simulink model "Noa_Nofusion_angle"  (R2020b)
settings: Solver=FixedStepDiscrete  StartTime=0.0  StopTime=Inf  FixedStep=0.01  RelTol=1e-3
PostLoadFcn:
  | if any(exist('dsrtsu_mdlpostloadfcn', 'file') ~= 0), dsrtsu_mdlpostloadfcn('Execute', bdroot); end
InitFcn:
  | , if any(exist('rtifpga_mdlclblib', 'file') ~= 0), rtifpga_mdlclblib('Init', bdroot); end,
  | , if any(exist('dsmpb_private', 'file') ~= 0), dsmpb_private('dsmpb_mdlclblib', 'Init', bdroot); end,
undefined symbols (not defined in the file): ACC_TimeGap_DecSetSwt, ACC_TimeGap_IncSetSwt, AccelPedalPosn, AccelPedalPosnVldty, AccelPedlPosnDiagc, AccPedalOverride, ACU_ShiftInProgress, ADAS_Posn_CurLane, AESSwtReq, ALC_SwtReq, BrkPedalSts, CC_ACC_CANCEL_OFFSwt, CC_ACC_CRUISE_OFFSwt, CC_ACC_DecSetSpd_SetSwt, CC_ACC_IncSetSpd_ResuSwt, CC_ACCSwtErr, CharSpd_ms, CSA_NODE, CURRENT_GEAR, CurrentGearValid, DiscIntNeverNeededParam, DrvDoorSts, DrvSBR, DrvTrqReqOvld, ECMACCInterface, ECMRespACC, ELKSwtReq, EngLimpHomeSts, EngSpd, EngState, EngState_PHEV, EngTrqMaxActSpd, EngTrqMinAct, EPS_DrvInpTrqVal_HighReslolution, EPS_FailSts, EPS_LKATorqOvrlDlvd, EPS_LKATorqOvrlDlvdVld, EPS_LKATrqOvlDlvdSts, EPS_SteerMod, EPS_TrqSnsrSts, EQ4_APPINFO, EQ4_LA_ELEM, EQ4_LA_HDR, EQ4_LAP_ELEM, EQ4_LAP_HDR, EQ4_LH_ELEM, EQ4_LH_HDR, EQ4_LRE_ELEM, EQ4_LRE_HDR, ESS_PedSwtReq, ESS_VehSwtReq, FFogLmpSts_F_Pbox, FLWheelDriveDirection, FLWheelSpd, FrntWiprSwtSts, FrntWshrSwtSts, FRWheelDriveDirection, FRWheelSpd, HazardLmpSwtSts, HCU_AccelPedalPosn_Diag ... (+151)
libraries: simulink x138, dsmpblib x33, canfdmsglib x10
(part 17 of 17)

== matlab function Noa_Nofusion_angle/TOS2/Subsystem1/ACCOSM/HWA_Task100ms1/ACC_DisplayBar ==
  data: TimeGap input; DisplayBar output uint8; DesireDistance input; ACCmode input; TargetRange input; Scale input; TargetExist input; DisplayBarK1 input uint8
function DisplayBar = fcn(TimeGap,DesireDistance,ACCmode,TargetRange,Scale,TargetExist,DisplayBarK1)
%#codegen
DisplayBar = DisplayBarK1;

ScaleDis = Scale*DesireDistance;
upScaleDis = (Scale+single(0.05))*DesireDistance;
lowScaleDis = (Scale-single(0.05))*DesireDistance;

i = TimeGap;

if (ACCmode==0)||(ACCmode==7)
    DisplayBar = uint8(0);
else
    if TargetExist==false
        DisplayBar=uint8(0);
    else
        switch(DisplayBarK1)
            case uint8(0)
                 if TargetRange> ScaleDis(i,3)
                     DisplayBar=uint8(4);
                 else
                     if TargetRange>ScaleDis(i,2)
                         DisplayBar=uint8(3);
                     else
                         if TargetRange>ScaleDis(i,1)
                             DisplayBar=uint8(2);
                         else
                             DisplayBar=uint8(1);
                         end
                     end
                 end
            case uint8(1)
                 if TargetRange> upScaleDis(i,3)
                     DisplayBar=uint8(4);
                 else
                     if TargetRange>upScaleDis(i,2)
                         DisplayBar=uint8(3);
                     else
                         if TargetRange>upScaleDis(i,1)
                             DisplayBar=uint8(2);
                         else
                             DisplayBar=uint8(1);
                         end
                     end
                 end
            case uint8(2)
                 if TargetRange> upScaleDis(i,3)
                     DisplayBar=uint8(4);
                 else
                     if TargetRange>upScaleDis(i,2)
                         DisplayBar=uint8(3);
                     else
                         if TargetRange>lowScaleDis(i,1)
                             DisplayBar=uint8(2);
                         else
                             DisplayBar=uint8(1);
                         end
                     end
                 end   
            case uint8(3)
                 if TargetRange> upScaleDis(i,3)
                     DisplayBar=uint8(4);
                 else
                     if TargetRange>lowScaleDis(i,2)
                         DisplayBar=uint8(3);
                     else
                         if TargetRange>lowScaleDis(i,1)
                             DisplayBar=uint8(2);
                         else
                             DisplayBar=uint8(1);
                         end
                     end
                end
            case uint8(4)
                 if TargetRange> lowScaleDis(i,3)
                     DisplayBar=uint8(4);
                 else
                     if TargetRange>lowScaleDis(i,2)
                         DisplayBar=uint8(3);
                     else
                         if TargetRange>lowScaleDis(i,1)
                             DisplayBar=uint8(2);
                         else
                             DisplayBar=uint8(1);
                         end
                     end
                 end      
        end    
    end
end

== matlab function Noa_Nofusion_angle/TOS2/Subsystem1/ACCOSM/HWA_Task100ms1/Dyc ==
  data: kapTrajFiltK1 input single size=1; vRef input single size=1; kapTrajFilt output single size=1; kapCourseErr output single; kapTraj input single size=1; alpSideSlipAngle input single size=1; A2 input single size=1; A1 input single size=1; LineValid input boolean size=1; ObjDx input single size=15; ObjDy input single size=15; TarLineValid input boolean; TarLineA2 input single; TarLineA1 input single; TarLineA0 input single size=1; dxC0 output single size=1; aPC0 output single size=1; bPC0 output single size=1; cPC0 output single size=1; aPC1 output single size=1; bPC1 output single size=1; cPC1 output single size=1; ObjDyc output single size=15
function [kapTrajFilt,kapCourseErr,dxC0,aPC0,bPC0,cPC0,aPC1,bPC1,cPC1,ObjDyc] = ...
    DriveCourseCalc(kapTrajFiltK1,vRef,kapTraj,alpSideSlipAngle,...
    A2,A1,LineValid,ObjDx,ObjDy,TarLineValid,TarLineA2,TarLineA1,TarLineA0)

ObjDyc = single(zeros(15,1));

if vRef>8.33
    t_alpSideSlipAngle = -alpSideSlipAngle;
else
    t_alpSideSlipAngle = single(0);
end

temp1 = single(0.1)/(single(0.1) + interpolate(single(24),single(0),single(55),single(0.4),vRef));

kapTrajFilt = kapTrajFiltK1 + temp1*(kapTraj - kapTrajFiltK1);

temp1 = abs(kapTraj*vRef);

if (temp1<0.001)&&(vRef>8.3)
    t_kapTrajwHyst = single(0);
else
    t_kapTrajwHyst = kapTrajFilt;
end

if TarLineValid
    temp = interpolate(single(0.2),single(0.2),single(1.5),single(1),abs(TarLineA0));
    dxC0Min = single(3);
else
    temp = single(1);
    dxC0Min = single(10);
end

dxC0 = max(vRef*temp,dxC0Min);
aPC0 = 0.5*t_kapTrajwHyst*(single(1)+1.5*t_alpSideSlipAngle*t_alpSideSlipAngle);
bPC0 = t_alpSideSlipAngle;
cPC0 = single(0);

temp1 = single(0.1)*abs(t_kapTrajwHyst);
temp2 = min(single(0.00013),single(0.004)/max(vRef,single(10)));
kapCourseErr = max(temp1,temp2);

aPC1 = aPC0;
bPC1 = bPC0;
cPC1 = single(0);

Low = interpolate(single(4),single(1),single(20),single(0),abs(atan(A1)));    % low vehiclespeed lanechange Angle is 4deg~20deg;
High = interpolate(single(4),single(1),single(10),single(0),abs(atan(A1)));   % low vehiclespeed lanechange Angle is 4deg~10deg;
t_vRefFactor = interpolate(single(5),Low,single(25),High,vRef);

t_Factor = single(1)*t_vRefFactor;

if TarLineValid==true
    aPC1 = TarLineA2;
    bPC1 = TarLineA1;
    cPC1 = (aPC0 - aPC1)*dxC0*dxC0 + (bPC0 - bPC1)*dxC0;
else
    if LineValid
        aPC1 = aPC0*(1 - t_Factor) + A2*t_Factor;
        bPC1 = bPC0*(1 - t_Factor) + A1*t_Factor;
        cPC1 = (aPC0 - aPC1)*dxC0*dxC0 + (bPC0 - bPC1)*dxC0;
    end
end

for i=1:15
   if ObjDx(i)>dxC0
      ObjDyc(i) =  ObjDy(i) - (aPC1*ObjDx(i)*ObjDx(i) + bPC1*ObjDx(i) + cPC1);
   else
      ObjDyc(i) =  ObjDy(i) - (aPC0*ObjDx(i)*ObjDx(i) + bPC0*ObjDx(i));
   end
end
end


function out = interpolate(x1,z1,x2,z2,Raw)
if Raw<=x1
    out = z1;
else
    if Raw>=x2
        out = z2;
    else
        out = z1 + (Raw-x1)*(z2-z1)/(x2-x1);
    end
end
end

== matlab function Noa_Nofusion_angle/TOS2/Subsystem1/ACCOSM/HWA_Task100ms1/DycCutIn ==
  data: ObjValid input boolean size=15; ObjDyc input single size=15; ObjMoveSts input uint8 size=15; ObjDycCutIn output single size=15; ObjMove_b output boolean size=15; ObjCnt input uint8 size=15; ObjDycHist input single size=15; ObjqDycHist input single size=15; dycFiltK1 input single size=15; ObjDycFilt output single size=15
function [ObjDycCutIn,ObjMove_b,ObjDycFilt] = ...
    ObjDycCutInCalc(ObjValid,ObjDyc,ObjMoveSts,ObjCnt,ObjDycHist,ObjqDycHist,dycFiltK1)
 
ObjDycCutIn = single(zeros(15,1));
ObjDycFilt = single(zeros(15,1));
ObjMove_b = false(15,1); 
 
for i=1:15
    if ObjValid(i)
        t_dyc = ObjDyc(i);
        t_dycHist = ObjDycHist(i);
        t_qDycHist = ObjqDycHist(i);
        
        weightDycHist = t_qDycHist*0.1;
        weightDyc = single(1) - weightDycHist;
        
        t_dycASI = weightDycHist*t_dycHist + weightDyc*t_dyc;
        ObjDycCutIn(i) = t_dycASI;
        
        if ObjCnt(i)>2
            ObjDycFilt(i) = 0.028*(t_dycASI - dycFiltK1(i)) + dycFiltK1(i);
        else
            ObjDycFilt(i) = t_dycASI;
        end
        if ObjMoveSts(i)==2
            ObjMove_b(i) = true;
        end
    end
end

== matlab function Noa_Nofusion_angle/TOS2/Subsystem1/ACCOSM/HWA_Task100ms1/DycHistCalc ==
  data: TrajHistBufferBTrajEnd input boolean; ObjTrajNumber input uint8; ObjDycHist output single; TrajCurrentIndex input uint8; TrajHistBufferBValid input boolean; TrajHistBufferDxv input single; TrajHistBufferDyv input single; ObjValid input boolean; ObjqDycHist output single; dxC0 input; aP0 input; bP0 input; cP0 input; aP1 input; bP1 input; cP1 input
function [ObjDycHist,ObjqDycHist] = DycHistCalc(TrajHistBufferBTrajEnd,ObjTrajNumber,TrajCurrentIndex,...
    TrajHistBufferBValid,TrajHistBufferDxv,TrajHistBufferDyv,ObjValid,dxC0,aP0,bP0,cP0,aP1,bP1,cP1)

t_dxv = single(0);
t_dyv = single(0);
t_dxvK1 = single(0);
t_dyvK1 = single(0);
ObjDycHist = single(zeros(15,1));
ObjqDycHist = single(zeros(15,1));

for iObj=1:15
    t_TrajNumber = ObjTrajNumber(iObj);
    if t_TrajNumber<21
        t_End = false;
        t_Failed = false;
        t_TrajCurrentIndex = TrajCurrentIndex(t_TrajNumber);
        t_TrajEnd = TrajHistBufferBTrajEnd(t_TrajNumber,t_TrajCurrentIndex);
        if (ObjValid(iObj)==true)&&(t_TrajEnd==false)
            for k=1:24
                if t_End==false
                    if t_TrajCurrentIndex<k
                        t_Index = t_TrajCurrentIndex + uint8(25) - k;
                    else
                        t_Index = t_TrajCurrentIndex - k + uint8(1);
                    end
                    if t_Index==1
                        t_IndexK1 = uint8(24);
                    else
                        t_IndexK1 = t_Index - uint8(1);
                    end
                    t_ValidK1 = TrajHistBufferBValid(t_TrajNumber,t_IndexK1);
                    t_TrajEndK1 = TrajHistBufferBTrajEnd(t_TrajNumber,t_IndexK1);
                    t_dxv = TrajHistBufferDxv(t_TrajNumber,t_Index);
                    t_dxvK1 = TrajHistBufferDxv(t_TrajNumber,t_IndexK1);
                    t_dyv = TrajHistBufferDyv(t_TrajNumber,t_Index);
                    t_dyvK1 = TrajHistBufferDyv(t_TrajNumber,t_IndexK1);
                    
                    if (t_TrajEndK1==true)||(t_ValidK1==false)
                        t_End = true;
                        t_Failed = true;
                    end
                    if (t_dxv>=0)&&(t_dxvK1<=0)
                        t_End = true;
                    end
                end
            end
        end
        if (t_End==true)&&(t_Failed==false)
            if (t_dxv==t_dxvK1)
                t_dycHist = t_dyv;
            else
                t_dycHist = t_dyv - t_dxv*(t_dyvK1 - t_dyv)/(t_dxvK1 - t_dxv);
            end
            t_qDycHist = single(1);  
        else
            if (t_End==true)&&(t_Failed==true)&&(t_dxv>0)
                if t_dxv>(dxC0)
                    t_dycHist = t_dyv - (aP1*t_dxv*t_dxv + bP1*t_dxv + cP1); 
                else
                    t_dycHist = t_dyv - (aP0*t_dxv*t_dxv + bP0*t_dxv + cP0); 
                end
               t_qDycHist = max((single(80) - t_dxv)/single(80),single(0));
            else
                t_dycHist = single(0);
                t_qDycHist = single(0);
            end
        end
    else
        t_dycHist = single(0);
        t_qDycHist = single(0);
    end
    ObjDycHist(iObj) = t_dycHist;
    ObjqDycHist(iObj) = t_qDycHist;
end

== matlab function Noa_Nofusion_angle/TOS2/Subsystem1/ACCOSM/HWA_Task100ms1/LostTargetCalc ==
  data: ObjValid input boolean size=15; ReID output uint8 size=1; ObjDx input single size=15; ObjDy input single size=15; DeltaDx input single size=1; DeltaDy input single size=1; P0IDK1 input uint8 size=1; P0VxK1 input single size=1; P0DxK1 input single size=1; P0DyK1 input single size=1; P0RangeK1 input; P0ArGK1 input; P0DycK1 input single size=1; P0VycK1 input single size=1; P0CutIn_bK1 input boolean size=1; tTargetLostK1 input single size=1; ReRange output single size=1; ReArG output single size=1; ReDx output single size=1; ReDy output single size=1; ReVx output single size=1; ReCutIn_b output boolean size=1; ReDyc output single size=1; ReVyc output single size=1; TargetLost_b output boolean size=1; Covered_b output boolean size=1; tTargetLost output single size=1
function [ReID,ReRange,ReArG,ReDx,ReDy,ReVx,ReCutIn_b,ReDyc,ReVyc,TargetLost_b,Covered_b,tTargetLost]...
    = LostTargetCalc(ObjValid,ObjDx,ObjDy,DeltaDx,DeltaDy,...
    P0IDK1,P0VxK1,P0DxK1,P0DyK1,P0RangeK1,P0ArGK1,P0DycK1,P0VycK1,P0CutIn_bK1,tTargetLostK1)
 
ReID = P0IDK1;
ReRange = single(255);
ReArG = single(0);
ReDx = single(255);
ReDy = single(0);
ReVx = single(0);
ReDyc = single(0);
ReVyc = single(0);
ReCutIn_b = false;
TargetLost_b = false;
tTargetLost = single(0);
Covered_b = false;
 
if (P0IDK1>0)&&(P0IDK1<100)    % k1 Exist Target
    if ObjValid(P0IDK1)==false
        ExistNearObj = false;
        P0DxPred = P0DxK1 + 0.1*P0VxK1;
        P0DyPred = P0DyK1;
        P0RangePred = P0RangeK1 + 0.1*P0VxK1; 
        for i=1:15
            if (ObjValid(i)==true)&&(ObjDx(i)<P0DxPred)
                Covered_b = CoveredCalc(P0DxPred,P0DyPred,ObjDx(i),ObjDy(i),single(2.1),single(-0.1));
                if Covered_b==true
                   break; 
                end
            end
            if (ObjValid(i)==1)&&(abs(ObjDx(i)-P0DxPred)<DeltaDx)&&(abs(ObjDy(i)-P0DyPred)<DeltaDy)
               ExistNearObj = true;
               ReID = uint8(i);
               ReDx = ObjDx(i);
            end
        end
        if (ExistNearObj==false)&&(Covered_b==false)
            TargetLost_b = true;
            tTargetLost = single(0.1);
            ReID = uint8(255);
            ReRange = P0RangePred;
            ReArG = P0ArGK1;
            ReDx = P0DxPred;
            ReDy = P0DyPred;
            ReVx = P0VxK1;
            ReCutIn_b = P0CutIn_bK1;
            ReVyc = P0VycK1;
            ReDyc = P0DycK1 + 0.1*P0VycK1;
        end
    end
else
    if P0IDK1>100   %  k1 Exist Target Re
        ExistNearObj = false;
        P0DxPred = P0DxK1 + 0.1*P0VxK1;
        P0DyPred = P0DyK1;
        P0RangePred = P0RangeK1 + 0.1*P0VxK1; 

        for i=1:15
            if (ObjValid(i)==1)&&(abs(ObjDx(i)-P0DxPred)<DeltaDx)&&(abs(ObjDy(i)-P0DyPred)<DeltaDy)
                ExistNearObj = true;
                ReID = uint8(i);
                ReDx = ObjDx(i);
                TargetLost_b = false;
                tTargetLost = single(0);
            end
        end
        if ExistNearObj==false
            TargetLost_b = true;
            tTargetLost = tTargetLostK1 + single(0.1);
            ReID = uint8(255);
            ReRange = P0RangePred;
            ReArG = P0ArGK1;
            ReDx = P0DxPred;
            ReDy = P0DyPred;
            ReVx = P0VxK1;
            ReCutIn_b = P0CutIn_bK1;
            ReVyc = P0VycK1;
            ReDyc = P0DycK1 + 0.1*P0VycK1;
        end
    end
end
end
 
function t_Covered_b = CoveredCalc(DxPred,DyPred,Dx,Dy,IFVDx,IFVDy)
y = (IFVDy - DyPred)*(Dx - DxPred)/(IFVDx - DxPred) + DyPred ;
Delta = single(0.8) + (Dx - IFVDx)/(DxPred - IFVDx);
if abs(Dy - y)<=Delta
    t_Covered_b = true;
else
    t_Covered_b = false;
end
end

== matlab function Noa_Nofusion_angle/TOS2/Subsystem1/ACCOSM/HWA_Task100ms1/Lpb ==
  data: vRef input single size=1; alpSumSlideCurveness input single size=1; ObjValid input boolean size=15; ObjDyc input single size=15; ObjLpb output single size=15; ObjDycHist input single size=15; ObjqDycHist input single size=15; ObjLpbL output single size=15; ObjLpbR output single size=15; ObjVyc input single size=15; ObjYawAngle input single size=15; ObjDylaneEdgeRight input; ObjDyEdgeWidthRight input; ObjDylaneEdgeLeft input; ObjDyEdgeWidthLeft input
function [ObjLpb,ObjLpbL,ObjLpbR] = LpbCalc(vRef,alpSumSlideCurveness,...
    ObjValid,ObjDyc,ObjDycHist,ObjqDycHist,ObjVyc,ObjYawAngle,...
    ObjDylaneEdgeRight,ObjDyEdgeWidthRight,ObjDylaneEdgeLeft,ObjDyEdgeWidthLeft)

 [ObjLpb,ObjLpbL,ObjLpbR] = LpbCalc(vRef,alpSumSlideCurveness,...
    ObjValid,ObjDyc,ObjDycHist,ObjqDycHist,ObjVyc,ObjYawAngle,...
    ObjDylaneEdgeRight,ObjDyEdgeWidthRight,ObjDylaneEdgeLeft,ObjDyEdgeWidthLeft);
end

== matlab function Noa_Nofusion_angle/TOS2/Subsystem1/ACCOSM/HWA_Task100ms1/OTL1/P0TrajHistCalc01 ==
  data: vRef input; tCycle input single; tSameHandle input single; CutIn input; P0Dx input single; P0Dy input single; P0TrajHistNum output uint8; EgoDDeltaX input single; EgoDDeltaY input single; EgoCosOfPsi input single; EgoSinOfPsi input single; P0TrajHistDxv output single; P0TrajHistDyv output single; P0TrajHistNumK1 input uint8; P0TrajHistDxvK1 input single; P0TrajHistDyvK1 input single
function [P0TrajHistNum,P0TrajHistDxv,P0TrajHistDyv]...
    = fcn(vRef, tCycle,tSameHandle,CutIn, P0Dx,P0Dy,EgoDDeltaX,EgoDDeltaY,EgoCosOfPsi,EgoSinOfPsi,...
    P0TrajHistNumK1,P0TrajHistDxvK1,P0TrajHistDyvK1)
%#codegen
P0TrajHistNum = P0TrajHistNumK1;
P0TrajHistDxv = P0TrajHistDxvK1;
P0TrajHistDyv = P0TrajHistDyvK1;

if tSameHandle==0
    P0TrajHistNum = uint8(0);
    P0TrajHistDxv = single(zeros(24,1));
    P0TrajHistDyv = single(zeros(24,1));
else
    if tSameHandle==tCycle
        if CutIn || (vRef>1)
            P0TrajHistDxv(1) = P0Dx;
            P0TrajHistDyv(1) = P0Dy;
            P0TrajHistNum = uint8(1);
        else
            P0TrajHistDxv(1) = P0Dx;
            P0TrajHistDyv(1) = P0Dy;
            P0TrajHistDxv(2) = P0Dx - single(1);
            P0TrajHistDyv(2) = P0Dy - single(1);
            P0TrajHistDxv(3) = P0Dx - single(2);
            P0TrajHistDyv(3) = P0Dy - single(2);
            P0TrajHistDxv(4) = P0Dx - single(3);
            P0TrajHistDyv(4) = P0Dy - single(3);
            P0TrajHistNum = uint8(4);
        end
    else
        Temp1 = P0TrajHistDxv(1) - EgoDDeltaX - P0Dx;
        Temp2 = P0TrajHistDyv(1) - EgoDDeltaY - P0Dy;
        dDeltaS = Temp1*Temp1 + Temp2*Temp2;
        
        t_d = interpolate(single(8),single(0.5),single(22),single(2.5),single(P0TrajHistNum));
        t_d = t_d*t_d;
        t_AddPosition = (dDeltaS>t_d);
        
        for iBuf=1:P0TrajHistNum
            dX = P0TrajHistDxv(iBuf)-EgoDDeltaX;
            dY = P0TrajHistDyv(iBuf)-EgoDDeltaY;
            P0TrajHistDxv(iBuf) = dX*EgoCosOfPsi + dY*EgoSinOfPsi;
            P0TrajHistDyv(iBuf) = -dX*EgoSinOfPsi + dY*EgoCosOfPsi;
            if (P0TrajHistDxv(iBuf)<-5)||(abs(P0TrajHistDyv(iBuf))>50)
                P0TrajHistNum = max(P0TrajHistNum - uint8(1),uint8(0));
            end
        end
        
        if t_AddPosition==true
            
            P0TrajHistNum = min(P0TrajHistNum + uint8(1),uint8(24));
            for iBuf= P0TrajHistNum:(-1):2
                P0TrajHistDxv(iBuf) = P0TrajHistDxv(iBuf-uint8(1));
                P0TrajHistDyv(iBuf) = P0TrajHistDyv(iBuf-uint8(1));
            end
            P0TrajHistDxv(1) = P0Dx;
            P0TrajHistDyv(1) = P0Dy;
        end
    end
end
end

function out = interpolate(x1,z1,x2,z2,Raw)
if Raw<=x1
    out = z1;
else
    if Raw>=x2
        out = z2;
    else
        out = z1 + (Raw-x1)*(z2-z1)/(x2-x1);
    end
end
end
